simulink model "SimulinkOnramp_Model_CruiseControl_Exercise2"  (R2024a)
settings: Solver=VariableStepAuto  StartTime=0.0  StopTime=10.0  RelTol=1e-3
StartFcn:
  | learning.simulink.modelCallbacks.startFunction(gcs)
StopFcn:
  | learning.simulink.modelCallbacks.stopFunction(gcs);
model workspace (MAT data in the model file):
  courseObject.course = 'simulink'
  courseObject.chapter = 2
  courseObject.lesson = 2
  courseObject.section = 1
  courseObject.task = 1
  t_ans = [0; 0.05; 0.1; 0.15; 0.2; 0.25; 0.3; 0.35; 0.4; 0.45; 0.5; 0.55; 0.6; 0.65; 0.7; 0.75; 0.8; 0.85; 0.9; 0.95; 1; 1; 1.05; 1.1; 1.15; 1.2; 1.25; 1.3; 1.35; 1.4; 1.45; 1.5; 1.55; 1.6; 1.65; 1.7; 1.75; 1.8; 1.85; 1.9; 1.95; 2; 2.05; 2.1; 2.15; 2.2; 2.25; 2.3; 2.35; 2.4; 2.45; 2.5; 2.55; 2.6; 2.65; 2.7; 2.75; 2.8; 2.85; 2.9; 2.95; 3; 3.05; 3.1; 3.15; 3.2; 3.25; 3.3; 3.35; 3.4; 3.45; 3.5; 3.55; 3.6; 3.65; 3.7; 3.75; 3.8; 3.85; 3.9; 3.95; 4; 4.05; 4.1; 4.15; 4.2; 4.25; 4.3; 4.35; 4.4; 4.45; 4.5; 4.55; 4.6; 4.65; 4.7; 4.75; 4.8; 4.85; 4.9; 4.95; 5; 5.05; 5.1; 5.15; 5.2; 5.25; 5.3; 5.35; 5.4; 5.45; 5.5; 5.55; 5.6; 5.65; 5.7; 5.75; 5.8; 5.85; 5.9; 5.95; 6; 6.05; 6.1; 6.15; 6.2; 6.25; 6.3; 6.35; 6.4; 6.45; 6.5; 6.55; 6.6; 6.65; 6.7; 6.75; 6.8; 6.85; 6.9; 6.95; 7; 7.05; 7.1; 7.15; 7.2; 7.25; 7.3; 7.35; 7.4; 7.45; 7.5; 7.55; 7.6; 7.65; 7.7; 7.75; 7.8; 7.85; 7.9; 7.95; 8; 8.05; 8.1; 8.15; 8.2; 8.25; 8.3; 8.35; 8.4; 8.45; 8.5; 8.55; 8.6; 8.65; 8.7; 8.75; 8.8; 8.85; 8.9; 8.95; 9; 9.05; 9.1; 9.15; 9.2; 9.25; 9.3; 9.35; 9.4; 9.45; 9.5; 9.55; 9.6; 9.65; 9.7; 9.75; 9.8; 9.85; 9.9; 9.95; 10]
  y_ans1 = [0 0 0 0 0 0 0 0 0 0 0 0 ... (202 elements, 202x1)]
libraries: slpidlib x1
CloseFcn:
  | learning.simulink.cleanupOnlineTraining;learning.simulink.Application.getInstance().dduxLogMatlabEvent("ModelClosed")
Description:
  | TrainingCourseModel
settings Model: Creator=ishans1  LastModifiedBy=ishans1
settings DataIOCC: SaveTime=off
settings RTWCC: GPUComputeCapability=3.5

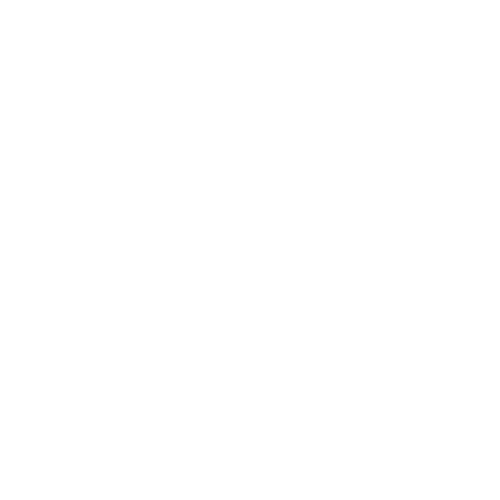
[thumbnail: Simulink's stored preview of the top-level diagram]
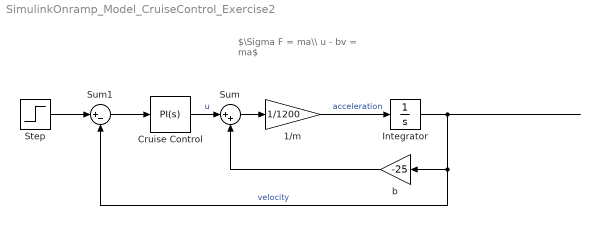
== system SimulinkOnramp_Model_CruiseControl_Exercise2 ==
  note: $\Sigma F = ma\\ u - bv = ma$
  1/m : Gain  Gain=1/1200
  Cruise Control : slpidlib/PID Controller  Controller=PI  Form=Parallel  TimeDomain=Continuous-time  UseExternalTs=off  SampleTime=-1  IntegratorMethod=Forward Euler  FilterMethod=Forward Euler  ControllerParametersSource=internal  P=1333.36349039677  I=31.1149911627912  UseKiTs=off  D=319.575242758411  UseExternalDerivativeSource=off  N=1  UseFilter=on  TunerSelectOption=Transfer Function Based (PID Tuner App)  InitialConditionSource=internal  InitialConditionForIntegrator=0  InitialConditionForFilter=0  DifferentiatorICPrevScaledInput=0  ExternalReset=none  TrackingMode=off  Kt=1  LimitOutput=off  SatLimitsSource=internal  UpperSaturationLimit=inf  LowerSaturationLimit=-inf  LinearizeAsGain=on  AntiWindupMode=none  Kb=1  LimitIntegrator=off  UpperIntegratorSaturationLimit=inf  LowerIntegratorSaturationLimit=-inf  POutMin=[]  POutMax=[]  IOutMin=[]  IOutMax=[]  DOutMin=[]  DOutMax=[]  NOutMin=[]  NOutMax=[]  SumOutMin=[]  SumOutMax=[]  SaturationOutMin=[]  SaturationOutMax=[]  PParamMin=[]  PParamMax=[]  IParamMin=[]  IParamMax=[]  DParamMin=[]  DParamMax=[]  NParamMin=[]  NParamMax=[]  KbParamMin=[]  KbParamMax=[]  KtParamMin=[]  KtParamMax=[]  KbOutMin=[]  KbOutMax=[]  KtOutMin=[]  KtOutMax=[]  IntegratorOutMin=[]  IntegratorOutMax=[]  FilterOutMin=[]  FilterOutMax=[]  SumI1OutMin=[]  SumI1OutMax=[]  SumI2OutMin=[]  SumI2OutMax=[]  SumI3OutMin=[]  SumI3OutMax=[]  SumI4OutMin=[]  SumI4OutMax=[]  SumDOutMin=[]  SumDOutMax=[]  DifferentiatorOutMin=[]  DifferentiatorOutMax=[]  FilterDiffOutCoefMin=[]  FilterDiffOutCoefMax=[]  ReciprocalOutMin=[]  ReciprocalOutMax=[]  SumDenOutMin=[]  SumDenOutMax=[]  SumNumOutMin=[]  SumNumOutMax=[]  DivideOutMin=[]  DivideOutMax=[]  UdiffTsProdOutMin=[]  UdiffTsProdOutMax=[]  NTsProdOutMin=[]  NTsProdOutMax=[]  UintegralTsProdOutMin=[]  UintegralTsProdOutMax=[]  UngainTsProdOutMin=[]  UngainTsProdOutMax=[]  ClampingZeroOutDataTypeStr=Inherit: Inherit via back propagation  ClampingZeroOutMin=[]  ClampingZeroOutMax=[]  FilterDenConstantOutDataTypeStr=Inherit: Inherit via back propagation  FilterDenConstantOutMin=[]  FilterDenConstantOutMax=[]  PCopyOutDataTypeStr=Inherit: Inherit via back propagation  PCopyOutMin=[]  PCopyOutMax=[]  NCopyOutDataTypeStr=Inherit: Inherit via back propagation  NCopyOutMin=[]  NCopyOutMax=[]  IntegratorContinuousStateAttributes=''  IntegratorStateMustResolveToSignalObject=off  IntegratorRTWStateStorageClass=Auto  FilterContinuousStateAttributes=''  FilterStateMustResolveToSignalObject=off  FilterRTWStateStorageClass=Auto  ParallelPVariant=InternalParameters  IdealPVariant=Disabled  IVariant=InternalParameters  DVariant=Disabled  IntegratorVariant=Continuous  SatVariant=Disabled  AWVariant=Passthrough  PCopyVariant=Disabled  TRVariant=Disabled  FdbkBlocksVariant=Forward  IdealPFdbkVariant=Disabled  SatFdbkVariant=Disabled  DerivativeFilterVariant=Disabled  NVariant=Disabled  NCopyVariant=Disabled_SignalSpec  FilterICVariant=Disabled  IntegratorICVariant=InternalICs  ExternalResetVariant=Disabled  TRSumVariant=Passthrough  SumFdbkVariant=Disabled  SumVariant=Sum_PI  TsampFilterVariant=InternalTs  TsampNgainVariant=Passthrough  TsampIntegralVariant=Disabled_SignalSpec  ExternalSaturationOutDataTypeStr=Inherit: Same as second input  DerivativeSourceVariant=Disabled
  Integrator : Integrator
  Step : Step  SampleTime=0
  Sum : Sum  Inputs=|++
  Sum1 : Sum  Inputs=|+-
  b : Gain  Gain=-25
  wires:
  b/1 -> Sum/2
  Sum1/1 -> Cruise Control/1
  Cruise Control/1 -> Sum/1  "u"
  Integrator/1 -> b/1, Sum1/2  "velocity"
  Sum/1 -> 1/m/1
  1/m/1 -> Integrator/1  "acceleration"
  Step/1 -> Sum1/1
